simulink model "softMBD_old"  (R2025b)
settings: Solver=FixedStepAuto  StartTime=0.0  StopTime=10  FixedStep=0.005  RelTol=1e-3
values from neighbouring files (symbols this model uses):
  FPV_mass = 0.8    [Soft.m]
  g = 9.81    [Soft.m]
  ks = 0    [Soft.m]
  p_0 = 1013.25    [Soft.m]
  Q2Ts = forcetomotors()    [Soft.m]    (also in forcetomotors.m = inv(Ts2Q))
  takeOffDuration = 2    [Soft.m]
  Ts = 0.005    [Soft.m]
undefined symbols (not defined in the file or in its folder): DiscIntNeverNeededParam, kd_pq, kd_pr, kd_y, ki_pq, ki_pr, ki_t, ki_y, kp_pq, kp_pr, kp_y, pInitialization
libraries: simulink x35, discretizing x11, slpidlib x2, shared6dof x1, dynamicsLibrary x1, aerolibasang x1, aerolibnav x1
(part 16 of 20)

== system softMBD_old/FCS/Controller/roll_pitch_controller/PID Controller/Anti-windup/Cont. Clamping Parallel ==
  preSat : Inport  SampleTime=SampleTime
  preInt : Inport  Port=2  SampleTime=SampleTime
  postSat : Inport  Port=3  SampleTime=SampleTime
  P : Inport  Port=4  SampleTime=SampleTime
  Upper Limit : Inport  Port=5  SampleTime=SampleTime
  Lower Limit : Inport  Port=6  SampleTime=SampleTime
  AND3 : Logic  DisableCoverage=on  OutDataTypeStr=boolean
  Constant1 : Constant  DisableCoverage=on  Value=0  OutDataTypeStr=Inherit: Inherit via back propagation  PreserveConstantTs=on
  DataTypeConv1 : DataTypeConversion  DisableCoverage=on  OutDataTypeStr=int8  SaturateOnIntegerOverflow=off  RndMeth=Floor
  DataTypeConv2 : DataTypeConversion  DisableCoverage=on  OutDataTypeStr=int8  SaturateOnIntegerOverflow=off  RndMeth=Floor
  Dead Zone : Subsystem  Variant=on  VariantControlMode=label  LabelModeActiveChoice=Disabled  EmptyChoice=on
  Equal1 : RelationalOperator  DisableCoverage=on  Operator===  OutDataTypeStr=boolean  RndMeth=Floor  InputSameDT=off
  Memory : Memory  DisableCoverage=on  InheritSampleTime=on
  NotEqual : RelationalOperator  DisableCoverage=on  Operator=~=  OutDataTypeStr=boolean  RndMeth=Floor  InputSameDT=off
  SignPreIntegrator : Signum  DisableCoverage=on
  SignPreSat : Signum  DisableCoverage=on
  Signal Specification2 : SignalSpecification  DisableCoverage=on  OutDataTypeStr=boolean  SampleTime=SampleTime
  Switch : Switch  Criteria=u2 > Threshold  SaturateOnIntegerOverflow=off
  Terminator1 : Terminator
  Terminator2 : Terminator
  ZeroGain : Gain  DisableCoverage=on  Gain=0  OutDataTypeStr=Inherit: Same as input  ParamDataTypeStr=Inherit: Same as input
  Out1 : Outport  SampleTime=SampleTime
  wires:
  Upper Limit/1 -> Dead Zone/2(Upper Limit)
  Lower Limit/1 -> Dead Zone/3(Lower Limit)
  AND3/1 -> Memory/1
  Constant1/1 -> Switch/1
  DataTypeConv2/1 -> Equal1/2
  DataTypeConv1/1 -> Equal1/1
  Equal1/1 -> AND3/2
  NotEqual/1 -> AND3/1
  SignPreIntegrator/1 -> DataTypeConv2/1
  SignPreSat/1 -> DataTypeConv1/1
  preInt/1 -> SignPreIntegrator/1, Switch/3
  Dead Zone/1(DZ out) -> SignPreSat/1, NotEqual/2
  ZeroGain/1 -> NotEqual/1
  preSat/1 -> ZeroGain/1, Dead Zone/1(preSat)
  Switch/1 -> Out1/1
  Memory/1 -> Switch/2
  Signal Specification2/1 -> Terminator2/1
  postSat/1 -> Terminator1/1
  P/1 -> Signal Specification2/1

== system softMBD_old/FCS/Controller/roll_pitch_controller/PID Controller/Anti-windup/Disabled ==
  preInt : Inport  SampleTime=SampleTime
  preSat : Inport  Port=2  SampleTime=SampleTime
  postSat : Inport  Port=3  SampleTime=SampleTime
  P : Inport  Port=4  SampleTime=SampleTime
  Signal Specification1 : SignalSpecification  DisableCoverage=on  OutDataTypeStr=boolean  SampleTime=SampleTime
  Signal Specification2 : SignalSpecification  DisableCoverage=on  OutDataTypeStr=boolean  SampleTime=SampleTime
  Terminator{,1..3} (4 alike) : Terminator
  wires:
  postSat/1 -> Terminator1/1
  Signal Specification2/1 -> Terminator2/1
  P/1 -> Signal Specification2/1
  preSat/1 -> Terminator/1
  preInt/1 -> Signal Specification1/1
  Signal Specification1/1 -> Terminator3/1

== system softMBD_old/FCS/Controller/roll_pitch_controller/PID Controller/Anti-windup/Disc. Clamping Ideal ==
  preSat : Inport  SampleTime=SampleTime
  P : Inport  Port=2  SampleTime=SampleTime
  preInt : Inport  Port=3  SampleTime=SampleTime
  postSat : Inport  Port=4  SampleTime=SampleTime
  Upper Limit : Inport  Port=5  SampleTime=SampleTime
  Lower Limit : Inport  Port=6  SampleTime=SampleTime
  AND1 : Logic  DisableCoverage=on  OutDataTypeStr=boolean
  AND2 : Logic  DisableCoverage=on  OutDataTypeStr=boolean
  AND3 : Logic  DisableCoverage=on  OutDataTypeStr=boolean
  Clamping_zero : Constant  DisableCoverage=on  Value=0  OutMin=ClampingZeroOutMin  OutMax=ClampingZeroOutMax  OutDataTypeStr=Inherit: Inherit via back propagation
  Constant1 : Constant  DisableCoverage=on  Value=0  OutDataTypeStr=Inherit: Inherit via back propagation  PreserveConstantTs=on
  Constant4 : Constant  DisableCoverage=on  OutDataTypeStr=int8
  Constant5 : Constant  DisableCoverage=on  Value=-1  OutDataTypeStr=int8
  Constant6 : Constant  DisableCoverage=on  OutDataTypeStr=int8
  Constant7 : Constant  DisableCoverage=on  Value=-1  OutDataTypeStr=int8
  Dead Zone : Subsystem  Variant=on  VariantControlMode=label  LabelModeActiveChoice=Disabled  EmptyChoice=on
  Equal1 : RelationalOperator  DisableCoverage=on  Operator===  OutDataTypeStr=boolean  RndMeth=Floor  InputSameDT=off
  NOT1 : Logic  DisableCoverage=on  Operator=NOT  OutDataTypeStr=boolean
  NOT2 : Logic  DisableCoverage=on  Operator=NOT  OutDataTypeStr=boolean
  OR1 : Logic  DisableCoverage=on  Operator=OR  OutDataTypeStr=boolean
  Relational Operator : RelationalOperator  DisableCoverage=on  Operator=~=  OutDataTypeStr=boolean  RndMeth=Simplest  InputSameDT=off
  Relational Operator1 : RelationalOperator  DisableCoverage=on  Operator=>  OutDataTypeStr=boolean  RndMeth=Simplest  InputSameDT=off
  Switch : Switch  Criteria=u2 > Threshold  SaturateOnIntegerOverflow=off
  Switch2 : Switch  DisableCoverage=on  Criteria=u2 > Threshold  SaturateOnIntegerOverflow=off  InputSameDT=off
  Switch3 : Switch  DisableCoverage=on  Criteria=u2 > Threshold  SaturateOnIntegerOverflow=off  InputSameDT=off
  Terminator1 : Terminator
  fix for DT propagation issue : RelationalOperator  DisableCoverage=on  Operator=>  OutDataTypeStr=boolean  RndMeth=Simplest  InputSameDT=off
  fix for DT propagation issue1 : RelationalOperator  DisableCoverage=on  Operator=>  OutDataTypeStr=boolean  RndMeth=Simplest  InputSameDT=off
  Out1 : Outport  SampleTime=SampleTime
  wires:
  fix for DT propagation issue1/1 -> Switch2/2
  P/1 -> Relational Operator1/1
  Relational Operator/1 -> AND3/1
  Dead Zone/1(DZ out) -> Relational Operator/2, fix for DT propagation issue/1
  fix for DT propagation issue/1 -> Switch3/2
  Clamping_zero/1 -> fix for DT propagation issue/2, fix for DT propagation issue1/2, Relational Operator1/2, Relational Operator/1
  Switch2/1 -> Equal1/2
  Switch3/1 -> Equal1/1
  Constant7/1 -> Switch3/3
  Constant6/1 -> Switch3/1
  Constant4/1 -> Switch2/1
  Constant5/1 -> Switch2/3
  Lower Limit/1 -> Dead Zone/3(Lower Limit)
  Upper Limit/1 -> Dead Zone/2(Upper Limit)
  Switch/1 -> Out1/1
  AND3/1 -> Switch/2
  Constant1/1 -> Switch/1
  OR1/1 -> AND3/2
  AND2/1 -> OR1/2
  AND1/1 -> OR1/1
  NOT2/1 -> AND2/2
  NOT1/1 -> AND2/1
  Relational Operator1/1 -> NOT2/1, AND1/2
  Equal1/1 -> AND1/1, NOT1/1
  preInt/1 -> fix for DT propagation issue1/1, Switch/3
  preSat/1 -> Dead Zone/1(preSat)
  postSat/1 -> Terminator1/1

== system softMBD_old/FCS/Controller/roll_pitch_controller/PID Controller/Anti-windup/Disc. Clamping Parallel ==
  preSat : Inport  SampleTime=SampleTime
  preInt : Inport  Port=2  SampleTime=SampleTime
  postSat : Inport  Port=3  SampleTime=SampleTime
  P : Inport  Port=4  SampleTime=SampleTime
  Upper Limit : Inport  Port=5  SampleTime=SampleTime
  Lower Limit : Inport  Port=6  SampleTime=SampleTime
  AND3 : Logic  DisableCoverage=on  OutDataTypeStr=boolean
  Clamping_zero : Constant  DisableCoverage=on  Value=0  OutMin=ClampingZeroOutMin  OutMax=ClampingZeroOutMax  OutDataTypeStr=Inherit: Inherit via back propagation
  Constant : Constant  DisableCoverage=on  OutDataTypeStr=int8
  Constant1 : Constant  DisableCoverage=on  Value=0  OutDataTypeStr=Inherit: Inherit via back propagation  PreserveConstantTs=on
  Constant2 : Constant  DisableCoverage=on  Value=-1  OutDataTypeStr=int8
  Constant3 : Constant  DisableCoverage=on  OutDataTypeStr=int8
  Constant4 : Constant  DisableCoverage=on  Value=-1  OutDataTypeStr=int8
  Dead Zone : Subsystem  Variant=on  VariantControlMode=label  LabelModeActiveChoice=Disabled  EmptyChoice=on
  Equal1 : RelationalOperator  DisableCoverage=on  Operator===  OutDataTypeStr=boolean  RndMeth=Floor  InputSameDT=off
  Relational Operator : RelationalOperator  DisableCoverage=on  Operator=~=  OutDataTypeStr=boolean  RndMeth=Simplest  InputSameDT=off
  Signal Specification2 : SignalSpecification  DisableCoverage=on  OutDataTypeStr=boolean  SampleTime=SampleTime
  Switch : Switch  Criteria=u2 > Threshold  SampleTime=SampleTime  SaturateOnIntegerOverflow=off
  Switch1 : Switch  DisableCoverage=on  Criteria=u2 > Threshold  SaturateOnIntegerOverflow=off  InputSameDT=off
  Switch2 : Switch  DisableCoverage=on  Criteria=u2 > Threshold  SaturateOnIntegerOverflow=off  InputSameDT=off
  Terminator1 : Terminator
  Terminator2 : Terminator
  fix for DT propagation issue : RelationalOperator  DisableCoverage=on  Operator=>  OutDataTypeStr=boolean  RndMeth=Simplest  InputSameDT=off
  fix for DT propagation issue1 : RelationalOperator  DisableCoverage=on  Operator=>  OutDataTypeStr=boolean  RndMeth=Simplest  InputSameDT=off
  Out1 : Outport  SampleTime=SampleTime
  wires:
  fix for DT propagation issue1/1 -> Switch2/2
  fix for DT propagation issue/1 -> Switch1/2
  Clamping_zero/1 -> fix for DT propagation issue/2, fix for DT propagation issue1/2, Relational Operator/1
  Constant1/1 -> Switch/1
  Switch2/1 -> Equal1/2
  Constant3/1 -> Switch2/1
  Constant4/1 -> Switch2/3
  Switch1/1 -> Equal1/1
  preInt/1 -> Switch/3, fix for DT propagation issue1/1
  Constant2/1 -> Switch1/3
  Constant/1 -> Switch1/1
  Relational Operator/1 -> AND3/1
  Lower Limit/1 -> Dead Zone/3(Lower Limit)
  Upper Limit/1 -> Dead Zone/2(Upper Limit)
  preSat/1 -> Dead Zone/1(preSat)
  Dead Zone/1(DZ out) -> Relational Operator/2, fix for DT propagation issue/1
  Equal1/1 -> AND3/2
  AND3/1 -> Switch/2
  Switch/1 -> Out1/1
  Signal Specification2/1 -> Terminator2/1
  postSat/1 -> Terminator1/1
  P/1 -> Signal Specification2/1

== system softMBD_old/FCS/Controller/roll_pitch_controller/PID Controller/Anti-windup/Passthrough ==
  preInt : Inport  SampleTime=SampleTime
  preSat : Inport  Port=2  SampleTime=SampleTime
  postSat : Inport  Port=3  SampleTime=SampleTime
  P : Inport  Port=4  SampleTime=SampleTime
  Signal Specification2 : SignalSpecification  DisableCoverage=on  OutDataTypeStr=boolean  SampleTime=SampleTime
  Terminator : Terminator
  Terminator1 : Terminator
  Terminator2 : Terminator
  Out1 : Outport  SampleTime=SampleTime
  wires:
  preInt/1 -> Out1/1
  preSat/1 -> Terminator/1
  postSat/1 -> Terminator1/1
  P/1 -> Signal Specification2/1
  Signal Specification2/1 -> Terminator2/1

== system softMBD_old/FCS/Controller/roll_pitch_controller/PID Controller/D Gain/Disabled ==
  D Gain : Inport  SampleTime=SampleTime
  Signal Specification : SignalSpecification  DisableCoverage=on  OutDataTypeStr=boolean  SampleTime=SampleTime
  Terminator : Terminator
  wires:
  D Gain/1 -> Signal Specification/1
  Signal Specification/1 -> Terminator/1

== system softMBD_old/FCS/Controller/roll_pitch_controller/PID Controller/D Gain/External Parameters ==
  err : Inport  SampleTime=SampleTime
  D Gain : Inport  Port=2  SampleTime=SampleTime
  DProd Out : Product  OutMin=DOutMin  OutMax=DOutMax  SampleTime=SampleTime
  Out1 : Outport  SampleTime=SampleTime
  wires:
  DProd Out/1 -> Out1/1
  D Gain/1 -> DProd Out/2
  err/1 -> DProd Out/1

== system softMBD_old/FCS/Controller/roll_pitch_controller/PID Controller/D Gain/Internal Parameters ==
  err : Inport  SampleTime=SampleTime
  D Gain : Inport  Port=2  SampleTime=SampleTime
  Derivative Gain : Gain  DisableCoverage=on  Gain=D  ParamMin=DParamMin  ParamMax=DParamMax  OutMin=DOutMin  OutMax=DOutMax
  Signal Specification : SignalSpecification  DisableCoverage=on  OutDataTypeStr=boolean  SampleTime=SampleTime
  Terminator : Terminator
  Out1 : Outport  SampleTime=SampleTime
  wires:
  Derivative Gain/1 -> Out1/1
  err/1 -> Derivative Gain/1
  D Gain/1 -> Signal Specification/1
  Signal Specification/1 -> Terminator/1

== system softMBD_old/FCS/Controller/roll_pitch_controller/PID Controller/External Derivative/Disabled ==
  ydot : Inport  SampleTime=SampleTime
  err : Inport  Port=2  SampleTime=SampleTime
  Signal Specification : SignalSpecification  DisableCoverage=on  OutDataTypeStr=boolean  SampleTime=SampleTime
  Terminator1 : Terminator
  Out1 : Outport  SampleTime=SampleTime
  wires:
  err/1 -> Terminator1/1
  Signal Specification/1 -> Out1/1
  ydot/1 -> Signal Specification/1

== system softMBD_old/FCS/Controller/roll_pitch_controller/PID Controller/External Derivative/Error ==
  err : Inport  SampleTime=SampleTime
  ydot : Inport  Port=2  SampleTime=SampleTime
  Signal Specification : SignalSpecification  DisableCoverage=on  OutDataTypeStr=boolean  SampleTime=SampleTime
  Terminator : Terminator
  Out1 : Outport  SampleTime=SampleTime
  wires:
  Signal Specification/1 -> Terminator/1
  ydot/1 -> Signal Specification/1
  err/1 -> Out1/1

== system softMBD_old/FCS/Controller/roll_pitch_controller/PID Controller/External Derivative/External Ydot ==
  err : Inport  SampleTime=SampleTime
  ydot : Inport  Port=2  SampleTime=SampleTime
  Terminator : Terminator
  Unary Minus : UnaryMinus
  Out1 : Outport  SampleTime=SampleTime
  wires:
  Unary Minus/1 -> Out1/1
  err/1 -> Terminator/1
  ydot/1 -> Unary Minus/1

== system softMBD_old/FCS/Controller/roll_pitch_controller/PID Controller/Filter/Cont. Filter ==
  U : Inport  SampleTime=SampleTime
  Nout : Inport  Port=2  SampleTime=SampleTime
  Reset : Inport  Port=3  SampleTime=SampleTime
  D0in : Inport  Port=4  SampleTime=SampleTime
  N : Inport  Port=5  SampleTime=SampleTime
  Ts : Inport  Port=6  SampleTime=SampleTime
  Filter : Integrator  DisableCoverage=on  InitialCondition=InitialConditionForFilter
  Signal Specification2 : SignalSpecification  DisableCoverage=on  OutDataTypeStr=boolean  SampleTime=SampleTime
  SumD : Sum  DisableCoverage=on  Inputs=|+-  OutMin=SumDOutMin  OutMax=SumDOutMax
  Terminator{,1..3} (4 alike) : Terminator
  Y : Outport  SampleTime=SampleTime
  wires:
  Ts/1 -> Terminator3/1
  D0in/1 -> Terminator/1
  U/1 -> SumD/1
  Filter/1 -> SumD/2
  SumD/1 -> Y/1
  Nout/1 -> Filter/1
  N/1 -> Signal Specification2/1
  Signal Specification2/1 -> Terminator2/1
  Reset/1 -> Terminator1/1

== system softMBD_old/FCS/Controller/roll_pitch_controller/PID Controller/Filter/Cont. Filter Only ==
  U : Inport  SampleTime=SampleTime
  Nout : Inport  Port=2  SampleTime=SampleTime
  Reset : Inport  Port=3  SampleTime=SampleTime
  D0in : Inport  Port=4  SampleTime=SampleTime
  N : Inport  Port=5  SampleTime=SampleTime
  Ts : Inport  Port=6  SampleTime=SampleTime
  Filter : Integrator  DisableCoverage=on  InitialCondition=InitialConditionForFilter
  Signal Specification2 : SignalSpecification  DisableCoverage=on  OutDataTypeStr=boolean  SampleTime=SampleTime
  SumD : Sum  DisableCoverage=on  Inputs=|+-  OutMin=SumDOutMin  OutMax=SumDOutMax
  Terminator{,1..3} (4 alike) : Terminator
  Y : Outport  SampleTime=SampleTime
  wires:
  Nout/1 -> SumD/2
  Filter/1 -> Y/1
  SumD/1 -> Filter/1
  Ts/1 -> Terminator3/1
  D0in/1 -> Terminator/1
  U/1 -> SumD/1
  N/1 -> Signal Specification2/1
  Signal Specification2/1 -> Terminator2/1
  Reset/1 -> Terminator1/1

== system softMBD_old/FCS/Controller/roll_pitch_controller/PID Controller/Filter/Differentiator ==
  U : Inport  SampleTime=SampleTime
  Reset : Inport  Port=2  SampleTime=SampleTime
  D0in : Inport  Port=3  SampleTime=SampleTime
  Nout : Inport  Port=4  SampleTime=SampleTime
  N : Inport  Port=5  SampleTime=SampleTime
  Ts : Inport  Port=6  SampleTime=SampleTime
  DTDup : DataTypeDuplicate  NumInputPorts=3
  Diff : Sum  Inputs=+-  OutMin=DifferentiatorOutMin  OutMax=DifferentiatorOutMax  OutDataTypeStr=Inherit: Inherit via back propagation  InputSameDT=on
  Signal Specification1 : SignalSpecification  DisableCoverage=on  OutDataTypeStr=boolean  SampleTime=SampleTime
  Terminator{,1..3} (4 alike) : Terminator
  Tsamp : Subsystem  Variant=on  VariantControlMode=label  LabelModeActiveChoice=InternalTs
  UD : Delay  DelayLength=1  InitialCondition=DifferentiatorICPrevScaledInput  SampleTime=SampleTime
  Y : Outport  OutMin=DifferentiatorOutMin  OutMax=DifferentiatorOutMax  SampleTime=SampleTime
  wires:
  Ts/1 -> Tsamp/2(Ts)
  D0in/1 -> Terminator/1
  U/1 -> Tsamp/1(U)
  UD/1 -> Diff/2, DTDup/3
  Tsamp/1(Out1) -> Diff/1, UD/1, DTDup/2
  Diff/1 -> Y/1, DTDup/1
  Nout/1 -> Terminator2/1
  N/1 -> Signal Specification1/1
  Signal Specification1/1 -> Terminator1/1
  Reset/1 -> Terminator3/1

== system softMBD_old/FCS/Controller/roll_pitch_controller/PID Controller/Filter/Disabled ==
  Reset : Inport  SampleTime=SampleTime
  U : Inport  Port=2  SampleTime=SampleTime
  N : Inport  Port=3  SampleTime=SampleTime
  D0in : Inport  Port=4  SampleTime=SampleTime
  Nout : Inport  Port=5  SampleTime=SampleTime
  Ts : Inport  Port=6  SampleTime=SampleTime
  Signal Specification{1..4} (4 alike) : SignalSpecification  DisableCoverage=on  OutDataTypeStr=boolean  SampleTime=SampleTime
  Terminator{1..6} (6 alike) : Terminator
  wires:
  Ts/1 -> Terminator6/1
  U/1 -> Signal Specification3/1
  Signal Specification3/1 -> Terminator3/1
  Signal Specification1/1 -> Terminator1/1
  N/1 -> Signal Specification1/1
  Nout/1 -> Signal Specification2/1
  Signal Specification4/1 -> Terminator4/1
  D0in/1 -> Signal Specification4/1
  Reset/1 -> Terminator5/1
  Signal Specification2/1 -> Terminator2/1

== system softMBD_old/FCS/Controller/roll_pitch_controller/PID Controller/Filter/Disc. Backward Euler Filter ==
  note: Denominator Coefficients
  U : Inport  SampleTime=SampleTime
  N : Inport  Port=2  SampleTime=SampleTime
  Reset : Inport  Port=3  SampleTime=SampleTime
  D0in : Inport  Port=4  SampleTime=SampleTime
  Nout : Inport  Port=5  SampleTime=SampleTime
  Ts : Inport  Port=6  SampleTime=SampleTime
  DenCoefOut : Product  OutMin=FilterDiffOutCoefMin  OutMax=FilterDiffOutCoefMax  SampleTime=SampleTime
  Filter Den Constant : Constant  DisableCoverage=on  OutMin=FilterDenConstantOutMin  OutMax=FilterDenConstantOutMax  OutDataTypeStr=Inherit: Inherit via back propagation  PreserveConstantTs=on
  Filter Differentiator TF : DiscreteTransferFcn  Numerator=[1 -1]  DenominatorSource=Input port  InitialStates=InitialConditionForFilter  SampleTime=SampleTime  a0EqualsOne=on
      settings: InputPortMap=u0,p3
  Mux : Mux  Inputs=2
  Passthrough for tuning : DataTypeConversion  Tag=#GainSurfaceTarget_  SaturateOnIntegerOverflow=off  RndMeth=Floor
  Reciprocal : Math  Operator=reciprocal  OutMin=ReciprocalOutMin  OutMax=ReciprocalOutMax  SaturateOnIntegerOverflow=off  OutDataTypeStr=Inherit: Inherit via internal rule
  SumDen : Sum  Inputs=++|  OutMin=SumDenOutMin  OutMax=SumDenOutMax  InputSameDT=on
  Terminator : Terminator
  Terminator1 : Terminator
  Terminator2 : Terminator
  Tsamp : Subsystem  Variant=on  VariantControlMode=label  LabelModeActiveChoice=InternalTs
  Unary Minus : UnaryMinus
  Y : Outport  SampleTime=SampleTime
  wires:
  Ts/1 -> Tsamp/2(Ts)
  D0in/1 -> Terminator/1
  Filter Differentiator TF/1 -> DenCoefOut/1
  DenCoefOut/1 -> Y/1
  U/1 -> Filter Differentiator TF/1
  Passthrough for tuning/1 -> Tsamp/1(N)
  N/1 -> Passthrough for tuning/1
  Filter Den Constant/1 -> SumDen/1, Mux/1
  Tsamp/1(Out1) -> SumDen/2
  Reciprocal/1 -> DenCoefOut/2, Unary Minus/1
  SumDen/1 -> Reciprocal/1
  Unary Minus/1 -> Mux/2
  Mux/1 -> Filter Differentiator TF/2
  Nout/1 -> Terminator2/1
  Reset/1 -> Terminator1/1

== system softMBD_old/FCS/Controller/roll_pitch_controller/PID Controller/Filter/Disc. Backward Euler Filter Only ==
  note: Denominator Coefficients
  U : Inport  SampleTime=SampleTime
  N : Inport  Port=2  SampleTime=SampleTime
  Reset : Inport  Port=3  SampleTime=SampleTime
  D0in : Inport  Port=4  SampleTime=SampleTime
  Nout : Inport  Port=5  SampleTime=SampleTime
  Ts : Inport  Port=6  SampleTime=SampleTime
  DenCoefOut : Product  OutMin=FilterDiffOutCoefMin  OutMax=FilterDiffOutCoefMax  SampleTime=SampleTime
  Filter Den Constant : Constant  DisableCoverage=on  OutMin=FilterDenConstantOutMin  OutMax=FilterDenConstantOutMax  OutDataTypeStr=Inherit: Inherit via back propagation  PreserveConstantTs=on
  Filter Differentiator TF : DiscreteTransferFcn  DenominatorSource=Input port  InitialStates=InitialConditionForFilter  SampleTime=SampleTime  a0EqualsOne=on
      settings: InputPortMap=u0,p3
  Mux : Mux  Inputs=2
  Passthrough for tuning : DataTypeConversion  Tag=#GainSurfaceTarget_  SaturateOnIntegerOverflow=off  RndMeth=Floor
  SumDen : Sum  Inputs=|++  OutMin=SumDenOutMin  OutMax=SumDenOutMax  InputSameDT=on
  Terminator : Terminator
  Terminator1 : Terminator
  Terminator2 : Terminator
  Tsamp : Subsystem  Variant=on  VariantControlMode=label  LabelModeActiveChoice=InternalTs
  Unary Minus : UnaryMinus
  Y : Outport  SampleTime=SampleTime
  wires:
  Filter Den Constant/1 -> Unary Minus/1, SumDen/2
  SumDen/1 -> Mux/1
  Unary Minus/1 -> Mux/2
  Reset/1 -> Terminator1/1
  Nout/1 -> Terminator2/1
  Mux/1 -> Filter Differentiator TF/2
  Tsamp/1(Out1) -> DenCoefOut/2, SumDen/1
  N/1 -> Passthrough for tuning/1
  Passthrough for tuning/1 -> Tsamp/1(N)
  U/1 -> Filter Differentiator TF/1
  DenCoefOut/1 -> Y/1
  Filter Differentiator TF/1 -> DenCoefOut/1
  D0in/1 -> Terminator/1
  Ts/1 -> Tsamp/2(Ts)

== system softMBD_old/FCS/Controller/roll_pitch_controller/PID Controller/Filter/Disc. Forward Euler Filter ==
  U : Inport  SampleTime=SampleTime
  Nout : Inport  Port=2  SampleTime=SampleTime
  Reset : Inport  Port=3  SampleTime=SampleTime
  D0in : Inport  Port=4  SampleTime=SampleTime
  N : Inport  Port=5  SampleTime=SampleTime
  Ts : Inport  Port=6  SampleTime=SampleTime
  Filter : DiscreteIntegrator  DisableCoverage=on  InitialCondition=InitialConditionForFilter  SampleTime=SampleTime  OutMin=FilterOutMin  OutMax=FilterOutMax  ICPrevOutput=DiscIntNeverNeededParam  ICPrevScaledInput=DiscIntNeverNeededParam
  Signal Specification2 : SignalSpecification  DisableCoverage=on  OutDataTypeStr=boolean  SampleTime=SampleTime
  SumD : Sum  DisableCoverage=on  Inputs=|+-  OutMin=SumDOutMin  OutMax=SumDOutMax
  Terminator{,1..3} (4 alike) : Terminator
  Y : Outport  SampleTime=SampleTime
  wires:
  Ts/1 -> Terminator3/1
  D0in/1 -> Terminator/1
  SumD/1 -> Y/1
  Nout/1 -> Filter/1
  U/1 -> SumD/1
  Filter/1 -> SumD/2
  N/1 -> Signal Specification2/1
  Signal Specification2/1 -> Terminator2/1
  Reset/1 -> Terminator1/1

== system softMBD_old/FCS/Controller/roll_pitch_controller/PID Controller/Filter/Disc. Forward Euler Filter Only ==
  U : Inport  SampleTime=SampleTime
  Nout : Inport  Port=2  SampleTime=SampleTime
  Reset : Inport  Port=3  SampleTime=SampleTime
  D0in : Inport  Port=4  SampleTime=SampleTime
  N : Inport  Port=5  SampleTime=SampleTime
  Ts : Inport  Port=6  SampleTime=SampleTime
  Filter : DiscreteIntegrator  DisableCoverage=on  InitialCondition=InitialConditionForFilter  SampleTime=SampleTime  OutMin=FilterOutMin  OutMax=FilterOutMax  ICPrevOutput=DiscIntNeverNeededParam  ICPrevScaledInput=DiscIntNeverNeededParam
  Signal Specification2 : SignalSpecification  DisableCoverage=on  OutDataTypeStr=boolean  SampleTime=SampleTime
  SumD : Sum  DisableCoverage=on  Inputs=|+-  OutMin=SumDOutMin  OutMax=SumDOutMax
  Terminator{,1..3} (4 alike) : Terminator
  Y : Outport  SampleTime=SampleTime
  wires:
  Filter/1 -> Y/1
  Reset/1 -> Terminator1/1
  Signal Specification2/1 -> Terminator2/1
  N/1 -> Signal Specification2/1
  Nout/1 -> SumD/2
  U/1 -> SumD/1
  SumD/1 -> Filter/1
  D0in/1 -> Terminator/1
  Ts/1 -> Terminator3/1

== system softMBD_old/FCS/Controller/roll_pitch_controller/PID Controller/Filter/Disc. Trapezoidal Filter ==
  note: Denominator Coefficients
  U : Inport  SampleTime=SampleTime
  N : Inport  Port=2  SampleTime=SampleTime
  Reset : Inport  Port=3  SampleTime=SampleTime
  D0in : Inport  Port=4  SampleTime=SampleTime
  Nout : Inport  Port=5  SampleTime=SampleTime
  Ts : Inport  Port=6  SampleTime=SampleTime
  DenCoefOut : Product  OutMin=FilterDiffOutCoefMin  OutMax=FilterDiffOutCoefMax  SampleTime=SampleTime
  Divide : Product  InputSameDT=on  OutMin=DivideOutMin  OutMax=DivideOutMax  SampleTime=SampleTime
  Filter Den Constant : Constant  DisableCoverage=on  OutMin=FilterDenConstantOutMin  OutMax=FilterDenConstantOutMax  OutDataTypeStr=Inherit: Inherit via back propagation  PreserveConstantTs=on
  Filter Differentiator TF : DiscreteTransferFcn  Numerator=[1 -1]  DenominatorSource=Input port  InitialStates=InitialConditionForFilter  SampleTime=SampleTime  a0EqualsOne=on
      settings: InputPortMap=u0,p3
  Mux : Mux  Inputs=2
  Passthrough for tuning : DataTypeConversion  Tag=#GainSurfaceTarget_  SaturateOnIntegerOverflow=off  RndMeth=Floor
  Reciprocal : Math  Operator=reciprocal  OutMin=ReciprocalOutMin  OutMax=ReciprocalOutMax  SaturateOnIntegerOverflow=off  OutDataTypeStr=Inherit: Inherit via internal rule
  SumDen : Sum  Inputs=++|  OutMin=SumDenOutMin  OutMax=SumDenOutMax  InputSameDT=on
  SumNum : Sum  Inputs=-+|  OutMin=SumNumOutMin  OutMax=SumNumOutMax  InputSameDT=on
  Terminator : Terminator
  Terminator1 : Terminator
  Terminator2 : Terminator
  Tsamp : Subsystem  Variant=on  VariantControlMode=label  LabelModeActiveChoice=InternalTs
  Y : Outport  SampleTime=SampleTime
  wires:
  Ts/1 -> Tsamp/2(Ts)
  D0in/1 -> Terminator/1
  Passthrough for tuning/1 -> Tsamp/1(N)
  Tsamp/1(Out1) -> SumDen/2, SumNum/2
  Filter Den Constant/1 -> SumNum/1, Mux/1, SumDen/1
  SumDen/1 -> Reciprocal/1
  SumNum/1 -> Divide/2
  Divide/1 -> Mux/2
  Reciprocal/1 -> DenCoefOut/2, Divide/1
  U/1 -> Filter Differentiator TF/1
  Filter Differentiator TF/1 -> DenCoefOut/1
  Mux/1 -> Filter Differentiator TF/2
  N/1 -> Passthrough for tuning/1
  DenCoefOut/1 -> Y/1
  Nout/1 -> Terminator2/1
  Reset/1 -> Terminator1/1

== system softMBD_old/FCS/Controller/roll_pitch_controller/PID Controller/Filter/Disc. Trapezoidal Filter Only ==
  note: Denominator Coefficients
  U : Inport  SampleTime=SampleTime
  N : Inport  Port=2  SampleTime=SampleTime
  Reset : Inport  Port=3  SampleTime=SampleTime
  D0in : Inport  Port=4  SampleTime=SampleTime
  Nout : Inport  Port=5  SampleTime=SampleTime
  Ts : Inport  Port=6  SampleTime=SampleTime
  DenCoefOut : Product  OutMin=FilterDiffOutCoefMin  OutMax=FilterDiffOutCoefMax  SampleTime=SampleTime
  Filter Den Constant : Constant  DisableCoverage=on  Value=2  OutMin=FilterDenConstantOutMin  OutMax=FilterDenConstantOutMax  OutDataTypeStr=Inherit: Inherit via back propagation  PreserveConstantTs=on
  Filter Differentiator TF : DiscreteTransferFcn  Numerator=[1 1]  DenominatorSource=Input port  InitialStates=InitialConditionForFilter  SampleTime=SampleTime  a0EqualsOne=on
      settings: InputPortMap=u0,p3
  Mux : Mux  Inputs=2
  Passthrough for tuning : DataTypeConversion  Tag=#GainSurfaceTarget_  SaturateOnIntegerOverflow=off  RndMeth=Floor
  SumDen : Sum  Inputs=|++  OutMin=SumDenOutMin  OutMax=SumDenOutMax  InputSameDT=on
  SumNum : Sum  Inputs=-+|  OutMin=SumNumOutMin  OutMax=SumNumOutMax  InputSameDT=on
  Terminator : Terminator
  Terminator1 : Terminator
  Terminator2 : Terminator
  Tsamp : Subsystem  Variant=on  VariantControlMode=label  LabelModeActiveChoice=InternalTs
  Y : Outport  SampleTime=SampleTime
  wires:
  SumNum/1 -> Mux/2
  SumDen/1 -> Mux/1
  Filter Den Constant/1 -> SumDen/1, SumNum/1
  Tsamp/1(Out1) -> SumDen/2, SumNum/2, DenCoefOut/2
  Reset/1 -> Terminator1/1
  Nout/1 -> Terminator2/1
  DenCoefOut/1 -> Y/1
  N/1 -> Passthrough for tuning/1
  Mux/1 -> Filter Differentiator TF/2
  Filter Differentiator TF/1 -> DenCoefOut/1
  U/1 -> Filter Differentiator TF/1
  Passthrough for tuning/1 -> Tsamp/1(N)
  D0in/1 -> Terminator/1
  Ts/1 -> Tsamp/2(Ts)

== system softMBD_old/FCS/Controller/roll_pitch_controller/PID Controller/Filter/Passthrough ==
  Reset : Inport  SampleTime=SampleTime
  U : Inport  Port=2  SampleTime=SampleTime
  N : Inport  Port=3  SampleTime=SampleTime
  D0in : Inport  Port=4  SampleTime=SampleTime
  Nout : Inport  Port=5  SampleTime=SampleTime
  Ts : Inport  Port=6  SampleTime=SampleTime
  Signal Specification1 : SignalSpecification  DisableCoverage=on  OutDataTypeStr=boolean  SampleTime=SampleTime
  Signal Specification4 : SignalSpecification  DisableCoverage=on  OutDataTypeStr=boolean  SampleTime=SampleTime
  Terminator{1..2,4..6} (5 alike) : Terminator
  Y : Outport  SampleTime=SampleTime
  wires:
  Nout/1 -> Terminator2/1
  Reset/1 -> Terminator5/1
  D0in/1 -> Signal Specification4/1
  Signal Specification4/1 -> Terminator4/1
  N/1 -> Signal Specification1/1
  Signal Specification1/1 -> Terminator1/1
  U/1 -> Y/1
  Ts/1 -> Terminator6/1

== system softMBD_old/FCS/Controller/roll_pitch_controller/PID Controller/Filter ICs/Disabled ==
  D0 : Inport  SampleTime=SampleTime
  Ground : Ground  DisableCoverage=on
  Signal Specification : SignalSpecification  DisableCoverage=on  OutDataTypeStr=boolean  SampleTime=SampleTime
  Signal Specification1 : SignalSpecification  DisableCoverage=on  OutDataTypeStr=boolean  SampleTime=SampleTime
  Terminator : Terminator
  Out1 : Outport  SampleTime=SampleTime
  wires:
  D0/1 -> Signal Specification/1
  Signal Specification/1 -> Terminator/1
  Ground/1 -> Signal Specification1/1
  Signal Specification1/1 -> Out1/1

== system softMBD_old/FCS/Controller/roll_pitch_controller/PID Controller/Filter ICs/External IC ==
  D0 : Inport  SampleTime=SampleTime
  Out1 : Outport  SampleTime=SampleTime
  wires:
  D0/1 -> Out1/1

== system softMBD_old/FCS/Controller/roll_pitch_controller/PID Controller/Filter ICs/Internal IC - Differentiator ==
  D0 : Inport  SampleTime=SampleTime
  Ground : Ground  DisableCoverage=on
  Signal Specification : SignalSpecification  DisableCoverage=on  OutDataTypeStr=boolean  SampleTime=SampleTime
  Signal Specification1 : SignalSpecification  DisableCoverage=on  OutDataTypeStr=boolean  SampleTime=SampleTime
  Terminator : Terminator
  Out1 : Outport  SampleTime=SampleTime
  wires:
  D0/1 -> Signal Specification/1
  Signal Specification/1 -> Terminator/1
  Ground/1 -> Signal Specification1/1
  Signal Specification1/1 -> Out1/1

== system softMBD_old/FCS/Controller/roll_pitch_controller/PID Controller/Filter ICs/Internal IC - Filter ==
  D0 : Inport  SampleTime=SampleTime
  Ground : Ground  DisableCoverage=on
  Signal Specification : SignalSpecification  DisableCoverage=on  OutDataTypeStr=boolean  SampleTime=SampleTime
  Signal Specification1 : SignalSpecification  DisableCoverage=on  OutDataTypeStr=boolean  SampleTime=SampleTime
  Terminator : Terminator
  Out1 : Outport  SampleTime=SampleTime
  wires:
  D0/1 -> Signal Specification/1
  Signal Specification/1 -> Terminator/1
  Ground/1 -> Signal Specification1/1
  Signal Specification1/1 -> Out1/1

== system softMBD_old/FCS/Controller/roll_pitch_controller/PID Controller/I Gain/Disabled ==
  I Gain : Inport  SampleTime=SampleTime
  Signal Specification : SignalSpecification  DisableCoverage=on  OutDataTypeStr=boolean  SampleTime=SampleTime
  Terminator : Terminator
  wires:
  Signal Specification/1 -> Terminator/1
  I Gain/1 -> Signal Specification/1

== system softMBD_old/FCS/Controller/roll_pitch_controller/PID Controller/I Gain/External Parameters ==
  err : Inport  SampleTime=SampleTime
  I Gain : Inport  Port=2  SampleTime=SampleTime
  IProd Out : Product  OutMin=IOutMin  OutMax=IOutMax  SampleTime=SampleTime
  Out1 : Outport  SampleTime=SampleTime
  wires:
  err/1 -> IProd Out/1
  I Gain/1 -> IProd Out/2
  IProd Out/1 -> Out1/1

== system softMBD_old/FCS/Controller/roll_pitch_controller/PID Controller/I Gain/Internal Parameters ==
  err : Inport  SampleTime=SampleTime
  I Gain : Inport  Port=2  SampleTime=SampleTime
  Integral Gain : Gain  DisableCoverage=on  Gain=I  ParamMin=IParamMin  ParamMax=IParamMax  OutMin=IOutMin  OutMax=IOutMax
  Signal Specification : SignalSpecification  DisableCoverage=on  OutDataTypeStr=boolean  SampleTime=SampleTime
  Terminator : Terminator
  Out1 : Outport  SampleTime=SampleTime
  wires:
  err/1 -> Integral Gain/1
  Integral Gain/1 -> Out1/1
  Signal Specification/1 -> Terminator/1
  I Gain/1 -> Signal Specification/1

== system softMBD_old/FCS/Controller/roll_pitch_controller/PID Controller/Ideal P Gain/External Parameters ==
  In1 : Inport  SampleTime=SampleTime
  P Gain : Inport  Port=2  SampleTime=SampleTime
  PProd Out : Product  SampleTime=SampleTime
  Out1 : Outport  SampleTime=SampleTime
  wires:
  In1/1 -> PProd Out/1
  P Gain/1 -> PProd Out/2
  PProd Out/1 -> Out1/1

== system softMBD_old/FCS/Controller/roll_pitch_controller/PID Controller/Ideal P Gain/Internal Parameters ==
  In1 : Inport  SampleTime=SampleTime
  P Gain : Inport  Port=2  SampleTime=SampleTime
  Proportional Gain : Gain  Gain=P  ParamMin=PParamMin  ParamMax=PParamMax  OutMin=POutMin  OutMax=POutMax
  Signal Specification1 : SignalSpecification  DisableCoverage=on  OutDataTypeStr=boolean  SampleTime=SampleTime
  Terminator1 : Terminator
  Out1 : Outport  SampleTime=SampleTime
  wires:
  In1/1 -> Proportional Gain/1
  Proportional Gain/1 -> Out1/1
  P Gain/1 -> Signal Specification1/1
  Signal Specification1/1 -> Terminator1/1

== system softMBD_old/FCS/Controller/roll_pitch_controller/PID Controller/Ideal P Gain/Passthrough ==
  In1 : Inport  SampleTime=SampleTime
  P Gain : Inport  Port=2  SampleTime=SampleTime
  Terminator1 : Terminator
  Out1 : Outport  SampleTime=SampleTime
  wires:
  In1/1 -> Out1/1
  P Gain/1 -> Terminator1/1

== system softMBD_old/FCS/Controller/roll_pitch_controller/PID Controller/Ideal P Gain Fdbk/Disabled ==
  In1 : Inport  SampleTime=SampleTime
  P Gain : Inport  Port=2  SampleTime=SampleTime
  Signal Specification1 : SignalSpecification  DisableCoverage=on  OutDataTypeStr=boolean  SampleTime=SampleTime
  Terminator1 : Terminator
  Terminator2 : Terminator
  wires:
  P Gain/1 -> Terminator1/1
  In1/1 -> Signal Specification1/1
  Signal Specification1/1 -> Terminator2/1

== system softMBD_old/FCS/Controller/roll_pitch_controller/PID Controller/Ideal P Gain Fdbk/External Parameters ==
  In1 : Inport  SampleTime=SampleTime
  P Gain : Inport  Port=2  SampleTime=SampleTime
  PProd Out : Product  SampleTime=SampleTime
  Out1 : Outport  SampleTime=SampleTime
  wires:
  PProd Out/1 -> Out1/1
  P Gain/1 -> PProd Out/2
  In1/1 -> PProd Out/1

== system softMBD_old/FCS/Controller/roll_pitch_controller/PID Controller/Ideal P Gain Fdbk/Internal Parameters ==
  In1 : Inport  SampleTime=SampleTime
  P Gain : Inport  Port=2  SampleTime=SampleTime
  Proportional Gain : Gain  Gain=P  ParamMin=PParamMin  ParamMax=PParamMax  OutMin=POutMin  OutMax=POutMax
  Signal Specification1 : SignalSpecification  DisableCoverage=on  OutDataTypeStr=boolean  SampleTime=SampleTime
  Terminator1 : Terminator
  Out1 : Outport  SampleTime=SampleTime
  wires:
  Proportional Gain/1 -> Out1/1
  In1/1 -> Proportional Gain/1
  Signal Specification1/1 -> Terminator1/1
  P Gain/1 -> Signal Specification1/1

== system softMBD_old/FCS/Controller/roll_pitch_controller/PID Controller/Ideal P Gain Fdbk/Passthrough ==
  In1 : Inport  SampleTime=SampleTime
  P Gain : Inport  Port=2  SampleTime=SampleTime
  Terminator1 : Terminator
  Out1 : Outport  SampleTime=SampleTime
  wires:
  In1/1 -> Out1/1
  P Gain/1 -> Terminator1/1

== system softMBD_old/FCS/Controller/roll_pitch_controller/PID Controller/Integrator/Continuous ==
  U : Inport  SampleTime=SampleTime
  Reset : Inport  Port=2  SampleTime=SampleTime
  I0in : Inport  Port=3  SampleTime=SampleTime
  Ground : Ground  DisableCoverage=on
  Integrator : Integrator  InitialCondition=InitialConditionForIntegrator  UpperSaturationLimit=UpperIntegratorSaturationLimit  LowerSaturationLimit=LowerIntegratorSaturationLimit
  Signal Specification1 : SignalSpecification  DisableCoverage=on  OutDataTypeStr=boolean  SampleTime=SampleTime
  Terminator : Terminator
  Terminator1 : Terminator
  state : Outport  SampleTime=SampleTime
  out : Outport  Port=2  SampleTime=SampleTime
  wires:
  U/1 -> Integrator/1
  I0in/1 -> Terminator/1
  Integrator/1 -> out/1
  Ground/1 -> Signal Specification1/1
  Signal Specification1/1 -> state/1
  Reset/1 -> Terminator1/1

== system softMBD_old/FCS/Controller/roll_pitch_controller/PID Controller/Integrator/Disabled ==
  U : Inport  SampleTime=SampleTime
  Reset : Inport  Port=2  SampleTime=SampleTime
  I0in : Inport  Port=3  SampleTime=SampleTime
  Ground : Ground  DisableCoverage=on
  Signal Specification1 : SignalSpecification  DisableCoverage=on  OutDataTypeStr=boolean  SampleTime=SampleTime
  Signal Specification2 : SignalSpecification  DisableCoverage=on  OutDataTypeStr=boolean  SampleTime=SampleTime
  Signal Specification4 : SignalSpecification  DisableCoverage=on  OutDataTypeStr=boolean  SampleTime=SampleTime
  Terminator1 : Terminator
  Terminator2 : Terminator
  Terminator3 : Terminator
  out : Outport  SampleTime=SampleTime
  wires:
  Reset/1 -> Terminator2/1
  Signal Specification4/1 -> Terminator1/1
  I0in/1 -> Signal Specification4/1
  U/1 -> Signal Specification1/1
  Signal Specification1/1 -> Terminator3/1
  Ground/1 -> Signal Specification2/1
  Signal Specification2/1 -> out/1

== system softMBD_old/FCS/Controller/roll_pitch_controller/PID Controller/Integrator/Discrete ==
  U : Inport  SampleTime=SampleTime
  Reset : Inport  Port=2  SampleTime=SampleTime
  I0in : Inport  Port=3  SampleTime=SampleTime
  Ground_Integrator : Ground  DisableCoverage=on
  Integrator : DiscreteIntegrator  InitialCondition=InitialConditionForIntegrator  SampleTime=SampleTime  OutMin=IntegratorOutMin  OutMax=IntegratorOutMax  UpperSaturationLimit=UpperIntegratorSaturationLimit  LowerSaturationLimit=LowerIntegratorSaturationLimit  ICPrevOutput=DiscIntNeverNeededParam  ICPrevScaledInput=DiscIntNeverNeededParam
  Signal Specification1 : SignalSpecification  DisableCoverage=on  OutDataTypeStr=boolean  SampleTime=SampleTime
  Terminator : Terminator
  Terminator1 : Terminator
  Terminator2 : Terminator
  out : Outport  SampleTime=SampleTime
  state : Outport  Port=2  SampleTime=SampleTime
  wires:
  I0in/1 -> Terminator1/1
  Integrator/1 -> out/1
  U/1 -> Integrator/1
  Ground_Integrator/1 -> state/1, Signal Specification1/1
  Signal Specification1/1 -> Terminator/1
  Reset/1 -> Terminator2/1

== system softMBD_old/FCS/Controller/roll_pitch_controller/PID Controller/Integrator ICs/Disabled ==
  I0 : Inport  SampleTime=SampleTime
  Ground : Ground  DisableCoverage=on
  Signal Specification : SignalSpecification  DisableCoverage=on  OutDataTypeStr=boolean  SampleTime=SampleTime
  Signal Specification1 : SignalSpecification  DisableCoverage=on  OutDataTypeStr=boolean  SampleTime=SampleTime
  Terminator : Terminator
  Out1 : Outport  SampleTime=SampleTime
  wires:
  Signal Specification/1 -> Terminator/1
  I0/1 -> Signal Specification/1
  Signal Specification1/1 -> Out1/1
  Ground/1 -> Signal Specification1/1

== system softMBD_old/FCS/Controller/roll_pitch_controller/PID Controller/Integrator ICs/External IC ==
  I0 : Inport  SampleTime=SampleTime
  Out1 : Outport  SampleTime=SampleTime
  wires:
  I0/1 -> Out1/1

== system softMBD_old/FCS/Controller/roll_pitch_controller/PID Controller/Integrator ICs/Internal IC ==
  I0 : Inport  SampleTime=SampleTime
  Ground : Ground  DisableCoverage=on
  Signal Specification : SignalSpecification  DisableCoverage=on  OutDataTypeStr=boolean  SampleTime=SampleTime
  Signal Specification1 : SignalSpecification  DisableCoverage=on  OutDataTypeStr=boolean  SampleTime=SampleTime
  Terminator : Terminator
  Out1 : Outport  SampleTime=SampleTime
  wires:
  I0/1 -> Signal Specification/1
  Signal Specification/1 -> Terminator/1
  Ground/1 -> Signal Specification1/1
  Signal Specification1/1 -> Out1/1

== system softMBD_old/FCS/Controller/roll_pitch_controller/PID Controller/N Copy/Disabled ==
  N Gain : Inport  SampleTime=SampleTime
  Terminator : Terminator
  wires:
  N Gain/1 -> Terminator/1

== system softMBD_old/FCS/Controller/roll_pitch_controller/PID Controller/N Copy/Disabled wSignal Specification ==
  N Gain : Inport  SampleTime=SampleTime
  Signal Specification1 : SignalSpecification  DisableCoverage=on  OutDataTypeStr=boolean  SampleTime=SampleTime
  Terminator : Terminator
  wires:
  N Gain/1 -> Signal Specification1/1
  Signal Specification1/1 -> Terminator/1

== system softMBD_old/FCS/Controller/roll_pitch_controller/PID Controller/N Copy/External Parameters ==
  N Gain : Inport  SampleTime=SampleTime
  Out1 : Outport  SampleTime=SampleTime
  wires:
  N Gain/1 -> Out1/1

== system softMBD_old/FCS/Controller/roll_pitch_controller/PID Controller/N Copy/Internal Parameters ==
  N Gain : Inport  SampleTime=SampleTime
  N Copy : Constant  DisableCoverage=on  Value=N  OutMin=NCopyOutMin  OutMax=NCopyOutMax  OutDataTypeStr=Inherit: Inherit via back propagation  PreserveConstantTs=on
  Signal Specification : SignalSpecification  DisableCoverage=on  OutDataTypeStr=boolean  SampleTime=SampleTime
  Terminator : Terminator
  Out1 : Outport  SampleTime=SampleTime
  wires:
  N Copy/1 -> Out1/1
  N Gain/1 -> Signal Specification/1
  Signal Specification/1 -> Terminator/1

== system softMBD_old/FCS/Controller/roll_pitch_controller/PID Controller/N Gain/Disabled ==
  U : Inport  SampleTime=SampleTime
  N Gain : Inport  Port=2  SampleTime=SampleTime
  Signal Specification1 : SignalSpecification  DisableCoverage=on  OutDataTypeStr=boolean  SampleTime=SampleTime
  Signal Specification2 : SignalSpecification  DisableCoverage=on  OutDataTypeStr=boolean  SampleTime=SampleTime
  Terminator1 : Terminator
  Terminator2 : Terminator
  wires:
  Signal Specification2/1 -> Terminator2/1
  U/1 -> Signal Specification2/1
  N Gain/1 -> Signal Specification1/1
  Signal Specification1/1 -> Terminator1/1

== system softMBD_old/FCS/Controller/roll_pitch_controller/PID Controller/N Gain/External Parameters ==
  U : Inport  SampleTime=SampleTime
  N Gain : Inport  Port=2  SampleTime=SampleTime
  NProd Out : Product  OutMin=NOutMin  OutMax=NOutMax  SampleTime=SampleTime
  Out1 : Outport  SampleTime=SampleTime
  wires:
  U/1 -> NProd Out/1
  N Gain/1 -> NProd Out/2
  NProd Out/1 -> Out1/1

== system softMBD_old/FCS/Controller/roll_pitch_controller/PID Controller/N Gain/Internal Parameters ==
  U : Inport  SampleTime=SampleTime
  N Gain : Inport  Port=2  SampleTime=SampleTime
  Filter Coefficient : Gain  Gain=N  ParamMin=NParamMin  ParamMax=NParamMax  OutMin=NOutMin  OutMax=NOutMax
  Signal Specification1 : SignalSpecification  DisableCoverage=on  OutDataTypeStr=boolean  SampleTime=SampleTime
  Terminator1 : Terminator
  Out1 : Outport  SampleTime=SampleTime
  wires:
  U/1 -> Filter Coefficient/1
  Filter Coefficient/1 -> Out1/1
  N Gain/1 -> Signal Specification1/1
  Signal Specification1/1 -> Terminator1/1

== system softMBD_old/FCS/Controller/roll_pitch_controller/PID Controller/N Gain/Passthrough ==
  U : Inport  SampleTime=SampleTime
  N Gain : Inport  Port=2  SampleTime=SampleTime
  Terminator1 : Terminator
  Out1 : Outport  SampleTime=SampleTime
  wires:
  U/1 -> Out1/1
  N Gain/1 -> Terminator1/1

== system softMBD_old/FCS/Controller/roll_pitch_controller/PID Controller/P Copy/Disabled ==
  P Gain : Inport  SampleTime=SampleTime
  Terminator3 : Terminator
  wires:
  P Gain/1 -> Terminator3/1

== system softMBD_old/FCS/Controller/roll_pitch_controller/PID Controller/P Copy/External Parameters Ideal ==
  P Gain : Inport  SampleTime=SampleTime
  Out1 : Outport  SampleTime=SampleTime
  wires:
  P Gain/1 -> Out1/1

== system softMBD_old/FCS/Controller/roll_pitch_controller/PID Controller/P Copy/Internal Parameters Ideal ==
  P Gain : Inport  SampleTime=SampleTime
  P Copy : Constant  DisableCoverage=on  Value=P  OutMin=PCopyOutMin  OutMax=PCopyOutMax  OutDataTypeStr=Inherit: Inherit via back propagation  PreserveConstantTs=on
  Terminator3 : Terminator
  Out1 : Outport  SampleTime=SampleTime
  wires:
  P Copy/1 -> Out1/1
  P Gain/1 -> Terminator3/1

== system softMBD_old/FCS/Controller/roll_pitch_controller/PID Controller/Parallel P Gain/Disabled ==
  P Gain : Inport  SampleTime=SampleTime
  Signal Specification : SignalSpecification  DisableCoverage=on  OutDataTypeStr=boolean  SampleTime=SampleTime
  Terminator : Terminator
  wires:
  P Gain/1 -> Signal Specification/1
  Signal Specification/1 -> Terminator/1

== system softMBD_old/FCS/Controller/roll_pitch_controller/PID Controller/Parallel P Gain/External Parameters ==
  err : Inport  SampleTime=SampleTime
  P Gain : Inport  Port=2  SampleTime=SampleTime
  PProd Out : Product  OutMin=POutMin  OutMax=POutMax  SampleTime=SampleTime
  Out1 : Outport  SampleTime=SampleTime
  wires:
  PProd Out/1 -> Out1/1
  P Gain/1 -> PProd Out/2
  err/1 -> PProd Out/1

== system softMBD_old/FCS/Controller/roll_pitch_controller/PID Controller/Parallel P Gain/Internal Parameters ==
  err : Inport  SampleTime=SampleTime
  P Gain : Inport  Port=2  SampleTime=SampleTime
  Proportional Gain : Gain  Gain=P  ParamMin=PParamMin  ParamMax=PParamMax  OutMin=POutMin  OutMax=POutMax
  Signal Specification : SignalSpecification  DisableCoverage=on  OutDataTypeStr=boolean  SampleTime=SampleTime
  Terminator : Terminator
  Out1 : Outport  SampleTime=SampleTime
  wires:
  Proportional Gain/1 -> Out1/1
  err/1 -> Proportional Gain/1
  Signal Specification/1 -> Terminator/1
  P Gain/1 -> Signal Specification/1

== system softMBD_old/FCS/Controller/roll_pitch_controller/PID Controller/Parallel P Gain/Passthrough ==
  err : Inport  SampleTime=SampleTime
  P Gain : Inport  Port=2  SampleTime=SampleTime
  Terminator : Terminator
  Out1 : Outport  SampleTime=SampleTime
  wires:
  err/1 -> Out1/1
  P Gain/1 -> Terminator/1

== system softMBD_old/FCS/Controller/roll_pitch_controller/PID Controller/Reset Signal/Disabled ==
  Reset : Inport  SampleTime=SampleTime
  Ground : Ground  DisableCoverage=on
  Signal Specification : SignalSpecification  DisableCoverage=on  OutDataTypeStr=boolean  SampleTime=SampleTime
  Signal Specification1 : SignalSpecification  DisableCoverage=on  OutDataTypeStr=boolean  SampleTime=SampleTime
  Terminator : Terminator
  Out1 : Outport  SampleTime=SampleTime
  wires:
  Reset/1 -> Signal Specification/1
  Signal Specification/1 -> Terminator/1
  Ground/1 -> Signal Specification1/1
  Signal Specification1/1 -> Out1/1

== system softMBD_old/FCS/Controller/roll_pitch_controller/PID Controller/Reset Signal/External Reset ==
  Reset : Inport  SampleTime=SampleTime
  Out1 : Outport  SampleTime=SampleTime
  wires:
  Reset/1 -> Out1/1

== system softMBD_old/FCS/Controller/roll_pitch_controller/PID Controller/Saturation/Enabled ==
  In1 : Inport  SampleTime=SampleTime
  Upper Limit : Inport  Port=2  SampleTime=SampleTime
  Lower Limit : Inport  Port=3  SampleTime=SampleTime
  Saturation : Saturate  UpperLimit=UpperSaturationLimit  LowerLimit=LowerSaturationLimit  SampleTime=SampleTime  OutMin=SaturationOutMin  OutMax=SaturationOutMax
  Signal Specification : SignalSpecification  DisableCoverage=on  OutDataTypeStr=boolean  SampleTime=SampleTime
  Signal Specification1 : SignalSpecification  DisableCoverage=on  OutDataTypeStr=boolean  SampleTime=SampleTime
  Terminator : Terminator
  Terminator1 : Terminator
  Out1 : Outport  SampleTime=SampleTime
  wires:
  Signal Specification1/1 -> Terminator1/1
  Upper Limit/1 -> Signal Specification/1
  Lower Limit/1 -> Signal Specification1/1
  Signal Specification/1 -> Terminator/1
  In1/1 -> Saturation/1
  Saturation/1 -> Out1/1

== system softMBD_old/FCS/Controller/roll_pitch_controller/PID Controller/Saturation/External ==
  In1 : Inport  SampleTime=SampleTime
  Upper Limit : Inport  Port=2  SampleTime=SampleTime
  Lower Limit : Inport  Port=3  SampleTime=SampleTime
  Saturation Dynamic : simulink/Discontinuities/Saturation Dynamic  OutMin=SaturationOutMin  OutMax=SaturationOutMax  OutDataTypeStr=Inherit: Same as second input  OutDataType=fixdt(1, 16)  OutScaling=2^-10  DoSatur=off
  Out1 : Outport  SampleTime=SampleTime
  wires:
  Lower Limit/1 -> Saturation Dynamic/3
  Upper Limit/1 -> Saturation Dynamic/1
  Saturation Dynamic/1 -> Out1/1
  In1/1 -> Saturation Dynamic/2

== system softMBD_old/FCS/Controller/roll_pitch_controller/PID Controller/Saturation/Passthrough ==
  In1 : Inport  SampleTime=SampleTime
  Upper Limit : Inport  Port=2  SampleTime=SampleTime
  Lower Limit : Inport  Port=3  SampleTime=SampleTime
  Signal Specification : SignalSpecification  DisableCoverage=on  OutDataTypeStr=boolean  SampleTime=SampleTime
  Signal Specification1 : SignalSpecification  DisableCoverage=on  OutDataTypeStr=boolean  SampleTime=SampleTime
  Terminator : Terminator
  Terminator1 : Terminator
  Out1 : Outport  SampleTime=SampleTime
  wires:
  Signal Specification1/1 -> Terminator1/1
  Lower Limit/1 -> Signal Specification1/1
  Upper Limit/1 -> Signal Specification/1
  Signal Specification/1 -> Terminator/1
  In1/1 -> Out1/1

== system softMBD_old/FCS/Controller/roll_pitch_controller/PID Controller/Saturation Fdbk/Disabled ==
  In1 : Inport  SampleTime=SampleTime
  Signal Specification1 : SignalSpecification  DisableCoverage=on  OutDataTypeStr=boolean  SampleTime=SampleTime
  Terminator1 : Terminator
  wires:
  In1/1 -> Signal Specification1/1
  Signal Specification1/1 -> Terminator1/1
